simulink model "DDCU_wxt_v02_forA_LabviewV02"  (R2014a)
settings: Solver=FixedStepDiscrete  StartTime=0.0  StopTime=50  FixedStep=0.0005  RelTol=1e-3
InitFcn:
  | Veh_Par_wxt
values from neighbouring files (symbols this model uses):
  ag_thr = 0.4*g    (= 3.924)    [Veh_Par_wxt.m]
  B = 2.25    [Veh_Par_wxt.m]
  bra_pre_em = 12    [Veh_Par_wxt.m]
  bra_pre_gz2 = 12/3    (= 4)    [Veh_Par_wxt.m]
  bra_pre_gz34 = 12/3    (= 4)    [Veh_Par_wxt.m]
  bra_pre_yd = 12/2    (= 6)    [Veh_Par_wxt.m]
  brakepre_dem_data = [0 1 2 3 4 5 6 7 8 9 10 11 12]    [Veh_Par_wxt.m]
  brakeTrq_dem_data = [0 218.198 436.396 654.594 872.792 1090.99 1309.188 1527.386 1745.584 1963.782 2181.98 2400.178 2618.376]    [Veh_Par_wxt.m]
  bratrq_max = 4*2618.376    (= 10473.504)    [Veh_Par_wxt.m]
  eff_tran = 0.75    [Veh_Par_wxt.m]
  G = Mass*g    (= 36297)    [Veh_Par_wxt.m]
  kd1 = 1    [Veh_Par_wxt.m]
  kd2 = 1    [Veh_Par_wxt.m]
  kd3 = 1    [Veh_Par_wxt.m]
  ki1 = 1    [Veh_Par_wxt.m]
  ki2 = 1    [Veh_Par_wxt.m]
  ki3 = 1    [Veh_Par_wxt.m]
  kp1 = 1    [Veh_Par_wxt.m]
  kp2 = 1    [Veh_Par_wxt.m]
  kp3 = 1    [Veh_Par_wxt.m]
  L = 3.12    [Veh_Par_wxt.m]
  premax = 12    [Veh_Par_wxt.m]
  Radius = 0.20    (= 0.2)    [Veh_Par_wxt.m]
  s_opt_yi_add = 0.05    [Veh_Par_wxt.m]
  s_opt_zhuan_add = 0.05    [Veh_Par_wxt.m]
  spd_map_mot = [0 100 200 300 360 400 500 600 700 800 900]*tras_ratio    [Veh_Par_wxt.m]
  spdmax = 900*tras_ratio    (= 5580)    [Veh_Par_wxt.m]
  speed_thr_park = 5/3.6/Radius*30/pi    (= 66.3145596216)    [Veh_Par_wxt.m]
  tras_ratio = 6.2    [Veh_Par_wxt.m]
  trq_map_mot = [1200 1200 1200 1200 1200 1080 864 720 617 540 480]/tras_ratio    [Veh_Par_wxt.m]
  trqmax = 80    [Veh_Par_wxt.m]
  v_thr1_b = 5    [Veh_Par_wxt.m]
  v_thr2_b = 20    [Veh_Par_wxt.m]
  v_thr_park = 5    [Veh_Par_wxt.m]
undefined symbols (not defined in the file or in its folder): DiscIntNeverNeededParam
libraries: simulink x231, ec5744lib x19
(part 3 of 16)

== system DDCU_wxt_v02_forA_LabviewV02/OutputSignalProcess/VCU_MCU2 ==
  M3Enable_in : Inport
  M3Mode_in : Inport  Port=2
  M3Drive_in : Inport  Port=3
  M3TorqueSet_in : Inport  Port=4
  M3SpeedLimit_in : Inport  Port=5
  M4Enable_in : Inport  Port=6
  M4Mode_in : Inport  Port=7
  M4Drive_in : Inport  Port=8
  M4TorqueSet_in : Inport  Port=9
  M4SpeedLimit_in : Inport  Port=10
  MCU2HeartBeat_in : Inport  Port=11
  Conv{1..8} (8 alike) : DataTypeConversion
  M3Drive : Subsystem
  M3Enable : Subsystem
  M3Mode : Subsystem
  M3SpeedLimit : Subsystem
  M3TorqueSet : Subsystem
  M4Drive : Subsystem
  M4Enable : Subsystem
  M4Mode : Subsystem
  M4SpeedLimit : Subsystem
  M4TorqueSet : Subsystem
  MCU2HeartBeat : Subsystem
  VCU_MCU2_DLC : Constant  Value=8  OutDataTypeStr=uint8
  VCU_MCU2_DLC_Out : Terminator
  VCU_MCU2_ID : Constant  Value=2348937218  OutDataTypeStr=single
  VCU_MCU2_ID_Out : Terminator
  VCU_MCU2_mux : Mux  Inputs=8
  or{1..8} (8 alike) : simulink/Logic and Bit Operations/Bitwise Operator  logicop=OR  UseBitMask=off  NumInputPorts=11  BitMask=bin2dec('11011001')  BitMaskRealWorld=Stored Integer
  output : Outport
  wires:
  VCU_MCU2_mux/1 -> output/1
  MCU2HeartBeat/1(output1) -> or1/1
  MCU2HeartBeat/2(output2) -> or2/1
  MCU2HeartBeat/3(output3) -> or3/1
  MCU2HeartBeat/4(output4) -> or4/1
  MCU2HeartBeat/5(output5) -> or5/1
  MCU2HeartBeat/6(output6) -> or6/1
  MCU2HeartBeat/7(output7) -> or7/1
  MCU2HeartBeat/8(output8) -> or8/1
  M4TorqueSet/1(output1) -> or1/2
  M4TorqueSet/2(output2) -> or2/2
  M4TorqueSet/3(output3) -> or3/2
  M4TorqueSet/4(output4) -> or4/2
  M4TorqueSet/5(output5) -> or5/2
  M4TorqueSet/6(output6) -> or6/2
  M4TorqueSet/7(output7) -> or7/2
  M4TorqueSet/8(output8) -> or8/2
  M4SpeedLimit/1(output1) -> or1/3
  M4SpeedLimit/2(output2) -> or2/3
  M4SpeedLimit/3(output3) -> or3/3
  M4SpeedLimit/4(output4) -> or4/3
  M4SpeedLimit/5(output5) -> or5/3
  M4SpeedLimit/6(output6) -> or6/3
  M4SpeedLimit/7(output7) -> or7/3
  M4SpeedLimit/8(output8) -> or8/3
  M4Mode/1(output1) -> or1/4
  M4Mode/2(output2) -> or2/4
  M4Mode/3(output3) -> or3/4
  M4Mode/4(output4) -> or4/4
  M4Mode/5(output5) -> or5/4
  M4Mode/6(output6) -> or6/4
  M4Mode/7(output7) -> or7/4
  M4Mode/8(output8) -> or8/4
  M4Enable/1(output1) -> or1/5
  M4Enable/2(output2) -> or2/5
  M4Enable/3(output3) -> or3/5
  M4Enable/4(output4) -> or4/5
  M4Enable/5(output5) -> or5/5
  M4Enable/6(output6) -> or6/5
  M4Enable/7(output7) -> or7/5
  M4Enable/8(output8) -> or8/5
  M4Drive/1(output1) -> or1/6
  M4Drive/2(output2) -> or2/6
  M4Drive/3(output3) -> or3/6
  M4Drive/4(output4) -> or4/6
  M4Drive/5(output5) -> or5/6
  M4Drive/6(output6) -> or6/6
  M4Drive/7(output7) -> or7/6
  M4Drive/8(output8) -> or8/6
  M3TorqueSet/1(output1) -> or1/7
  M3TorqueSet/2(output2) -> or2/7
  M3TorqueSet/3(output3) -> or3/7
  M3TorqueSet/4(output4) -> or4/7
  M3TorqueSet/5(output5) -> or5/7
  M3TorqueSet/6(output6) -> or6/7
  M3TorqueSet/7(output7) -> or7/7
  M3TorqueSet/8(output8) -> or8/7
  M3SpeedLimit/1(output1) -> or1/8
  M3SpeedLimit/2(output2) -> or2/8
  M3SpeedLimit/3(output3) -> or3/8
  M3SpeedLimit/4(output4) -> or4/8
  M3SpeedLimit/5(output5) -> or5/8
  M3SpeedLimit/6(output6) -> or6/8
  M3SpeedLimit/7(output7) -> or7/8
  M3SpeedLimit/8(output8) -> or8/8
  M3Mode/1(output1) -> or1/9
  M3Mode/2(output2) -> or2/9
  M3Mode/3(output3) -> or3/9
  M3Mode/4(output4) -> or4/9
  M3Mode/5(output5) -> or5/9
  M3Mode/6(output6) -> or6/9
  M3Mode/7(output7) -> or7/9
  M3Mode/8(output8) -> or8/9
  M3Enable/1(output1) -> or1/10
  M3Enable/2(output2) -> or2/10
  M3Enable/3(output3) -> or3/10
  M3Enable/4(output4) -> or4/10
  M3Enable/5(output5) -> or5/10
  M3Enable/6(output6) -> or6/10
  M3Enable/7(output7) -> or7/10
  M3Enable/8(output8) -> or8/10
  M3Drive/1(output1) -> or1/11
  M3Drive/2(output2) -> or2/11
  M3Drive/3(output3) -> or3/11
  M3Drive/4(output4) -> or4/11
  M3Drive/5(output5) -> or5/11
  M3Drive/6(output6) -> or6/11
  M3Drive/7(output7) -> or7/11
  M3Drive/8(output8) -> or8/11
  or1/1 -> Conv1/1
  Conv1/1 -> VCU_MCU2_mux/1
  or2/1 -> Conv2/1
  Conv2/1 -> VCU_MCU2_mux/2
  or3/1 -> Conv3/1
  Conv3/1 -> VCU_MCU2_mux/3
  or4/1 -> Conv4/1
  Conv4/1 -> VCU_MCU2_mux/4
  or5/1 -> Conv5/1
  Conv5/1 -> VCU_MCU2_mux/5
  or6/1 -> Conv6/1
  Conv6/1 -> VCU_MCU2_mux/6
  or7/1 -> Conv7/1
  Conv7/1 -> VCU_MCU2_mux/7
  or8/1 -> Conv8/1
  Conv8/1 -> VCU_MCU2_mux/8
  VCU_MCU2_ID/1 -> VCU_MCU2_ID_Out/1
  VCU_MCU2_DLC/1 -> VCU_MCU2_DLC_Out/1
  MCU2HeartBeat_in/1 -> MCU2HeartBeat/1(MCU2HeartBeat)
  M4TorqueSet_in/1 -> M4TorqueSet/1(M4TorqueSet)
  M4SpeedLimit_in/1 -> M4SpeedLimit/1(M4SpeedLimit)
  M4Mode_in/1 -> M4Mode/1(M4Mode)
  M4Enable_in/1 -> M4Enable/1(M4Enable)
  M4Drive_in/1 -> M4Drive/1(M4Drive)
  M3TorqueSet_in/1 -> M3TorqueSet/1(M3TorqueSet)
  M3SpeedLimit_in/1 -> M3SpeedLimit/1(M3SpeedLimit)
  M3Mode_in/1 -> M3Mode/1(M3Mode)
  M3Enable_in/1 -> M3Enable/1(M3Enable)
  M3Drive_in/1 -> M3Drive/1(M3Drive)

== matlab function DDCU_wxt_v02_forA_LabviewV02/MainControl/mode_control/forward/forward/Drive/驱动防滑控制TCS/转向TCS/左转/前轮滑转/HeartBeat ==
  data: life_pre input; life output
function life = fcn(life_pre)
%#codegen
life=life_pre+1;
if life>15
    life=0;
end
end

== matlab function DDCU_wxt_v02_forA_LabviewV02/MainControl/mode_control/forward/forward/Drive/驱动防滑控制TCS/转向TCS/左转/后轮滑转/HeartBeat ==
  data: life_pre input; life output
function life = fcn(life_pre)
%#codegen
life=life_pre+1;
if life>15
    life=0;
end
end

== matlab function DDCU_wxt_v02_forA_LabviewV02/MainControl/mode_control/forward/forward/Drive/驱动防滑控制TCS/转向TCS/左转/前后轮均滑转/HeartBeat ==
  data: life_pre input; life output
function life = fcn(life_pre)
%#codegen
life=life_pre+1;
if life>15
    life=0;
end
end

== matlab function DDCU_wxt_v02_forA_LabviewV02/MainControl/mode_control/forward/forward/Drive/驱动防滑控制TCS/转向TCS/右转/MATLAB Function1 ==
  data: s_act_lr input; flag_lr output; s_opt_zhuan input; s_opt_zhuan_add input; flag_lr_pre input
function flag_lr = fcn(s_act_lr,s_opt_zhuan,s_opt_zhuan_add,flag_lr_pre)
%#codegen
if s_act_lr>s_opt_zhuan+s_opt_zhuan_add
    flag_lr=1;
elseif s_act_lr<s_opt_zhuan
    flag_lr = 0;
else
    flag_lr=flag_lr_pre;
end
end

== matlab function DDCU_wxt_v02_forA_LabviewV02/MainControl/mode_control/forward/forward/Drive/驱动防滑控制TCS/转向TCS/右转/MATLAB Function4 ==
  data: y output; flag_lf input; flag_lr input
function y = fcn(flag_lf,flag_lr)
%#codegen只判断外侧车轮滑转状况，不能满足要求再进一步修改。
if flag_lf==0 && flag_lr==0
    y=0;
elseif flag_lf==1 && flag_lr==0
    y=1;
elseif flag_lf==0 && flag_lr==1
    y=2;
else
    %     flag_lf==1 && flag_lr==1
    y=3;
end
end

== matlab function DDCU_wxt_v02_forA_LabviewV02/MainControl/mode_control/forward/forward/Drive/驱动防滑控制TCS/转向TCS/右转/后轮滑转/HeartBeat1 ==
  data: life_pre input; life output
function life = fcn(life_pre)
%#codegen
life=life_pre+1;
if life>15
    life=0;
end
end

== matlab function DDCU_wxt_v02_forA_LabviewV02/MainControl/mode_control/forward/forward/Drive/驱动防滑控制TCS/转向TCS/右转/无滑转/HeartBeat ==
  data: life_pre input; life output
function life = fcn(life_pre)
%#codegen
life=life_pre+1;
if life>15
    life=0;
end
end

== matlab function DDCU_wxt_v02_forA_LabviewV02/MainControl/mode_control/neutral/neutral/HeartBeat ==
  data: life_pre input; life output
function life = fcn(life_pre)
%#codegen
life=life_pre+1;
if life>15
    life=0;
end
end

== matlab function DDCU_wxt_v02_forA_LabviewV02/MainControl/mode_control/forward/forward/Brake/MATLAB Function2 ==
  data: syi_act_lr input; flagyi_lr output; s_opt_yi input; s_opt_yi_add input; flagyi_lr_pre input
function flagyi_lr = fcn(syi_act_lr,s_opt_yi,s_opt_yi_add,flagyi_lr_pre)
%#codegen
if syi_act_lr>s_opt_yi+s_opt_yi_add
    flagyi_lr=1;
elseif syi_act_lr<s_opt_yi
    flagyi_lr = 0;
else
    flagyi_lr=flagyi_lr_pre;
end
end

== matlab function DDCU_wxt_v02_forA_LabviewV02/MainControl/mode_control/forward/forward/Brake/HeartBeat ==
  data: life_pre input; life output
function life = fcn(life_pre)
%#codegen
life=life_pre+1;
if life>15
    life=0;
end
end

== matlab function DDCU_wxt_v02_forA_LabviewV02/MainControl/mode_control/center_steer/center_steer/容错控制/MATLAB Function ==
  data: trq_dem_l input; trq_dem_lf output; trq_dem_r input; trqlim_lf input; trqlim_lr input; trqlim_rf input; trqlim_rr input; guzhang_lf input; guzhang_lr input; guzhang_rf input; guzhang_rr input; trq_dem_lr output; trq_dem_rf output; trq_dem_rr output; bra_pre_l output; bra_pre_r output; bra_pre_yd input; mode output
function [trq_dem_lf,trq_dem_lr,trq_dem_rf,trq_dem_rr,bra_pre_l,bra_pre_r,mode] = fcn(trq_dem_l,trq_dem_r,trqlim_lf,trqlim_lr,trqlim_rf,trqlim_rr,guzhang_lf,guzhang_lr,guzhang_rf,guzhang_rr,bra_pre_yd)
%#codegen
if guzhang_lf==0 && guzhang_lr==0 && guzhang_rf==0 && guzhang_rr==0    %0电机故障,平均分配
    trq_dem_lf=trq_dem_l/2;
    trq_dem_lr=trq_dem_l/2;
    trq_dem_rf=trq_dem_r/2;
    trq_dem_rr=trq_dem_r/2;
    bra_pre_l=0;
    bra_pre_r=0;
    mode=1;
elseif  guzhang_lf==1 && guzhang_lr==0 && guzhang_rf==0 && guzhang_rr==0  %1电机故障，同侧电机进行力矩转移,跟行车不同，对侧不降扭。
    trq_dem_lf=0;
    trq_dem_lr=min(trq_dem_l,trqlim_lr);
    trq_dem_rf=trq_dem_r/2;
    trq_dem_rr=trq_dem_r/2;
    bra_pre_l=0;
    bra_pre_r=0;
    mode=2;
elseif  guzhang_lf==0 && guzhang_lr==1 && guzhang_rf==0 && guzhang_rr==0
    trq_dem_lf=min(trq_dem_l,trqlim_lf);
    trq_dem_lr=0;
    trq_dem_rf=trq_dem_r/2;
    trq_dem_rr=trq_dem_r/2;
    bra_pre_l=0;
    bra_pre_r=0;
    mode=3;
elseif  guzhang_lf==0 && guzhang_lr==0 && guzhang_rf==1 && guzhang_rr==0
    trq_dem_rf=0;
    trq_dem_rr=min(trq_dem_r,trqlim_rr);
    trq_dem_lf=trq_dem_l/2;
    trq_dem_lr=trq_dem_l/2;
    bra_pre_l=0;
    bra_pre_r=0;
    mode=4;
elseif  guzhang_lf==0 && guzhang_lr==0 && guzhang_rf==0 && guzhang_rr==1
    trq_dem_rf=min(trq_dem_r,trqlim_rf);
    trq_dem_rr=0;
    trq_dem_lf=trq_dem_l/2;
    trq_dem_lr=trq_dem_l/2;
    bra_pre_l=0;
    bra_pre_r=0;
    mode=5;
elseif  guzhang_lf==1 && guzhang_lr==1 && guzhang_rf==0 && guzhang_rr==0  %2电机故障，左侧双电机故障，左侧履带施加制动，改为原地转向
    trq_dem_lf=0;
    trq_dem_lr=0;
    trq_dem_rf=trq_dem_r/2;
    trq_dem_rr=trq_dem_r/2;
    bra_pre_l=bra_pre_yd;
    bra_pre_r=0;
    mode=6;
elseif  guzhang_lf==0 && guzhang_lr==0 && guzhang_rf==1 && guzhang_rr==1  %右侧双电机故障
    trq_dem_lf=trq_dem_l/2;
    trq_dem_lr=trq_dem_l/2;
    trq_dem_rf=0;
    trq_dem_rr=0;
    bra_pre_l=0;
    bra_pre_r=bra_pre_yd;
    mode=7;
elseif  guzhang_lf==1 && guzhang_lr==0 && guzhang_rf==1 && guzhang_rr==0 %2电机故障，对侧双电机故障,有4种情况,前两电机故障
    trq_dem_lf=0;
    trq_dem_rf=0;
    trq_dem_lr=min(trq_dem_l,trqlim_lr);
    trq_dem_rr=min(trq_dem_r,trqlim_rr);
    bra_pre_l=0;
    bra_pre_r=0;
    mode=8;
elseif  guzhang_lf==0 && guzhang_lr==1 && guzhang_rf==0 && guzhang_rr==1 %后两电机故障
    trq_dem_lr=0;
    trq_dem_rr=0;
    trq_dem_lf=min(trq_dem_l,trqlim_lf);
    trq_dem_rf=min(trq_dem_r,trqlim_rf);
    bra_pre_l=0;
    bra_pre_r=0;
    mode=9;
elseif  guzhang_lf==1 && guzhang_lr==0 && guzhang_rf==0 && guzhang_rr==1 %左前电机和右后电机故障
    trq_dem_lf=0;
    trq_dem_rr=0;
    trq_dem_lr=min(trq_dem_l,trqlim_lr);
    trq_dem_rf=min(trq_dem_r,trqlim_rf);
    bra_pre_l=0;
    bra_pre_r=0;
    mode=10;
elseif  guzhang_lf==0 && guzhang_lr==1 && guzhang_rf==1 && guzhang_rr==0 %左后电机和右前电机故障
    trq_dem_lr=0;
    trq_dem_rf=0;
    trq_dem_lf=min(trq_dem_l,trqlim_lf);
    trq_dem_rr=min(trq_dem_r,trqlim_rr);
    bra_pre_l=0;
    bra_pre_r=0;
    mode=11;
elseif guzhang_lf==1 && guzhang_lr==1 && guzhang_rf==1 && guzhang_rr==0   % 三电机故障
    trq_dem_lf=0;
    trq_dem_lr=0;
    trq_dem_rf=0;
    trq_dem_rr=min(trq_dem_r,trqlim_rr);
    bra_pre_l=bra_pre_yd;
    bra_pre_r=0;
    mode=12;
elseif guzhang_lf==1 && guzhang_lr==1 && guzhang_rf==0 && guzhang_rr==1
    trq_dem_lf=0;
    trq_dem_lr=0;
    trq_dem_rf=min(trq_dem_r,trqlim_rf);
    trq_dem_rr=0;
    bra_pre_l=bra_pre_yd;
    bra_pre_r=0;
    mode=13;
elseif guzhang_lf==1 && guzhang_lr==0 && guzhang_rf==1 && guzhang_rr==1
    trq_dem_lf=0;
    trq_dem_lr=min(trq_dem_l,trqlim_lr);
    trq_dem_rf=0;
    trq_dem_rr=0;
    bra_pre_l=0;
    bra_pre_r=bra_pre_yd;
    mode=14;
elseif guzhang_lf==0 && guzhang_lr==1 && guzhang_rf==1 && guzhang_rr==1
    trq_dem_lf=min(trq_dem_l,trqlim_lf);
    trq_dem_lr=0;
    trq_dem_rf=0;
    trq_dem_rr=0;
    bra_pre_l=0;
    bra_pre_r=bra_pre_yd;
    mode=15;
else
    %     guzhang_lf==1 && guzhang_lr==1 && guzhang_rf==1 && guzhang_rr==1 %四电机故障
    trq_dem_lf=0;
    trq_dem_lr=0;
    trq_dem_rf=0;
    trq_dem_rr=0;
    bra_pre_l=0;
    bra_pre_r=0;
    mode=16;
end
trq_dem_lf=min(trqlim_lf,trq_dem_lf);trq_dem_lf=max(0,trq_dem_lf);
trq_dem_lr=min(trqlim_lr,trq_dem_lr);trq_dem_lr=max(0,trq_dem_lr);
trq_dem_rf=min(trqlim_rf,trq_dem_rf);trq_dem_rf=max(0,trq_dem_rf);
trq_dem_rr=min(trqlim_rr,trq_dem_rr);trq_dem_rr=max(0,trq_dem_rr);
bra_pre_l=bra_pre_l;
bra_pre_r=bra_pre_r;
end

== system DDCU_wxt_v02_forA_LabviewV02/OutputSignalProcess/VCU_MCU2_replace ==
  M4SpeedSet_in : Inport
  M3SpeedSet_in : Inport  Port=2
  MCU2HeartBeat_in : Inport  Port=3
  M4SpeedLimit_in : Inport  Port=4
  M4Mode_in : Inport  Port=5
  M4Enable_in : Inport  Port=6
  M4Drive_in : Inport  Port=7
  M3SpeedLimit_in : Inport  Port=8
  M3Mode_in : Inport  Port=9
  M3Enable_in : Inport  Port=10
  M3Drive_in : Inport  Port=11
  Conv{1..8} (8 alike) : DataTypeConversion
  M3Drive : Subsystem
  M3Enable : Subsystem
  M3Mode : Subsystem
  M3SpeedLimit : Subsystem
  M3SpeedSet : Subsystem
  M4Drive : Subsystem
  M4Enable : Subsystem
  M4Mode : Subsystem
  M4SpeedLimit : Subsystem
  M4SpeedSet : Subsystem
  MCU2HeartBeat : Subsystem
  VCU_MCU2_replace_DLC : Constant  Value=8  OutDataTypeStr=uint8
  VCU_MCU2_replace_DLC_Out : Terminator
  VCU_MCU2_replace_ID : Constant  Value=2348937234  OutDataTypeStr=single
  VCU_MCU2_replace_ID_Out : Terminator
  VCU_MCU2_replace_mux : Mux  Inputs=8
  or{1..8} (8 alike) : simulink/Logic and Bit Operations/Bitwise Operator  logicop=OR  UseBitMask=off  NumInputPorts=11  BitMask=bin2dec('11011001')  BitMaskRealWorld=Stored Integer
  output : Outport
  wires:
  VCU_MCU2_replace_mux/1 -> output/1
  M4SpeedSet/1(output1) -> or1/1
  M4SpeedSet/2(output2) -> or2/1
  M4SpeedSet/3(output3) -> or3/1
  M4SpeedSet/4(output4) -> or4/1
  M4SpeedSet/5(output5) -> or5/1
  M4SpeedSet/6(output6) -> or6/1
  M4SpeedSet/7(output7) -> or7/1
  M4SpeedSet/8(output8) -> or8/1
  M3SpeedSet/1(output1) -> or1/2
  M3SpeedSet/2(output2) -> or2/2
  M3SpeedSet/3(output3) -> or3/2
  M3SpeedSet/4(output4) -> or4/2
  M3SpeedSet/5(output5) -> or5/2
  M3SpeedSet/6(output6) -> or6/2
  M3SpeedSet/7(output7) -> or7/2
  M3SpeedSet/8(output8) -> or8/2
  MCU2HeartBeat/1(output1) -> or1/3
  MCU2HeartBeat/2(output2) -> or2/3
  MCU2HeartBeat/3(output3) -> or3/3
  MCU2HeartBeat/4(output4) -> or4/3
  MCU2HeartBeat/5(output5) -> or5/3
  MCU2HeartBeat/6(output6) -> or6/3
  MCU2HeartBeat/7(output7) -> or7/3
  MCU2HeartBeat/8(output8) -> or8/3
  M4SpeedLimit/1(output1) -> or1/4
  M4SpeedLimit/2(output2) -> or2/4
  M4SpeedLimit/3(output3) -> or3/4
  M4SpeedLimit/4(output4) -> or4/4
  M4SpeedLimit/5(output5) -> or5/4
  M4SpeedLimit/6(output6) -> or6/4
  M4SpeedLimit/7(output7) -> or7/4
  M4SpeedLimit/8(output8) -> or8/4
  M4Mode/1(output1) -> or1/5
  M4Mode/2(output2) -> or2/5
  M4Mode/3(output3) -> or3/5
  M4Mode/4(output4) -> or4/5
  M4Mode/5(output5) -> or5/5
  M4Mode/6(output6) -> or6/5
  M4Mode/7(output7) -> or7/5
  M4Mode/8(output8) -> or8/5
  M4Enable/1(output1) -> or1/6
  M4Enable/2(output2) -> or2/6
  M4Enable/3(output3) -> or3/6
  M4Enable/4(output4) -> or4/6
  M4Enable/5(output5) -> or5/6
  M4Enable/6(output6) -> or6/6
  M4Enable/7(output7) -> or7/6
  M4Enable/8(output8) -> or8/6
  M4Drive/1(output1) -> or1/7
  M4Drive/2(output2) -> or2/7
  M4Drive/3(output3) -> or3/7
  M4Drive/4(output4) -> or4/7
  M4Drive/5(output5) -> or5/7
  M4Drive/6(output6) -> or6/7
  M4Drive/7(output7) -> or7/7
  M4Drive/8(output8) -> or8/7
  M3SpeedLimit/1(output1) -> or1/8
  M3SpeedLimit/2(output2) -> or2/8
  M3SpeedLimit/3(output3) -> or3/8
  M3SpeedLimit/4(output4) -> or4/8
  M3SpeedLimit/5(output5) -> or5/8
  M3SpeedLimit/6(output6) -> or6/8
  M3SpeedLimit/7(output7) -> or7/8
  M3SpeedLimit/8(output8) -> or8/8
  M3Mode/1(output1) -> or1/9
  M3Mode/2(output2) -> or2/9
  M3Mode/3(output3) -> or3/9
  M3Mode/4(output4) -> or4/9
  M3Mode/5(output5) -> or5/9
  M3Mode/6(output6) -> or6/9
  M3Mode/7(output7) -> or7/9
  M3Mode/8(output8) -> or8/9
  M3Enable/1(output1) -> or1/10
  M3Enable/2(output2) -> or2/10
  M3Enable/3(output3) -> or3/10
  M3Enable/4(output4) -> or4/10
  M3Enable/5(output5) -> or5/10
  M3Enable/6(output6) -> or6/10
  M3Enable/7(output7) -> or7/10
  M3Enable/8(output8) -> or8/10
  M3Drive/1(output1) -> or1/11
  M3Drive/2(output2) -> or2/11
  M3Drive/3(output3) -> or3/11
  M3Drive/4(output4) -> or4/11
  M3Drive/5(output5) -> or5/11
  M3Drive/6(output6) -> or6/11
  M3Drive/7(output7) -> or7/11
  M3Drive/8(output8) -> or8/11
  or1/1 -> Conv1/1
  Conv1/1 -> VCU_MCU2_replace_mux/1
  or2/1 -> Conv2/1
  Conv2/1 -> VCU_MCU2_replace_mux/2
  or3/1 -> Conv3/1
  Conv3/1 -> VCU_MCU2_replace_mux/3
  or4/1 -> Conv4/1
  Conv4/1 -> VCU_MCU2_replace_mux/4
  or5/1 -> Conv5/1
  Conv5/1 -> VCU_MCU2_replace_mux/5
  or6/1 -> Conv6/1
  Conv6/1 -> VCU_MCU2_replace_mux/6
  or7/1 -> Conv7/1
  Conv7/1 -> VCU_MCU2_replace_mux/7
  or8/1 -> Conv8/1
  Conv8/1 -> VCU_MCU2_replace_mux/8
  VCU_MCU2_replace_ID/1 -> VCU_MCU2_replace_ID_Out/1
  VCU_MCU2_replace_DLC/1 -> VCU_MCU2_replace_DLC_Out/1
  M4SpeedSet_in/1 -> M4SpeedSet/1(M4SpeedSet)
  M3SpeedSet_in/1 -> M3SpeedSet/1(M3SpeedSet)
  MCU2HeartBeat_in/1 -> MCU2HeartBeat/1(MCU2HeartBeat)
  M4SpeedLimit_in/1 -> M4SpeedLimit/1(M4SpeedLimit)
  M4Mode_in/1 -> M4Mode/1(M4Mode)
  M4Enable_in/1 -> M4Enable/1(M4Enable)
  M4Drive_in/1 -> M4Drive/1(M4Drive)
  M3SpeedLimit_in/1 -> M3SpeedLimit/1(M3SpeedLimit)
  M3Mode_in/1 -> M3Mode/1(M3Mode)
  M3Enable_in/1 -> M3Enable/1(M3Enable)
  M3Drive_in/1 -> M3Drive/1(M3Drive)

== system DDCU_wxt_v02_forA_LabviewV02/OutputSignalProcess/VCU_Park ==
  ParkEnable_in : Inport
  Conv{1..8} (8 alike) : DataTypeConversion
  ParkEnable : Subsystem
  VCU_Park_DLC : Constant  Value=8  OutDataTypeStr=uint8
  VCU_Park_DLC_Out : Terminator
  VCU_Park_ID : Constant  Value=2281988666  OutDataTypeStr=single
  VCU_Park_ID_Out : Terminator
  VCU_Park_mux : Mux  Inputs=8
  or{1..8} (8 alike) : simulink/Logic and Bit Operations/Bitwise Operator  logicop=OR  UseBitMask=off  BitMask=bin2dec('11011001')  BitMaskRealWorld=Stored Integer
  output : Outport
  wires:
  VCU_Park_mux/1 -> output/1
  ParkEnable/1(output1) -> or1/1
  ParkEnable/2(output2) -> or2/1
  ParkEnable/3(output3) -> or3/1
  ParkEnable/4(output4) -> or4/1
  ParkEnable/5(output5) -> or5/1
  ParkEnable/6(output6) -> or6/1
  ParkEnable/7(output7) -> or7/1
  ParkEnable/8(output8) -> or8/1
  or1/1 -> Conv1/1
  Conv1/1 -> VCU_Park_mux/1
  or2/1 -> Conv2/1
  Conv2/1 -> VCU_Park_mux/2
  or3/1 -> Conv3/1
  Conv3/1 -> VCU_Park_mux/3
  or4/1 -> Conv4/1
  Conv4/1 -> VCU_Park_mux/4
  or5/1 -> Conv5/1
  Conv5/1 -> VCU_Park_mux/5
  or6/1 -> Conv6/1
  Conv6/1 -> VCU_Park_mux/6
  or7/1 -> Conv7/1
  Conv7/1 -> VCU_Park_mux/7
  or8/1 -> Conv8/1
  Conv8/1 -> VCU_Park_mux/8
  VCU_Park_ID/1 -> VCU_Park_ID_Out/1
  VCU_Park_DLC/1 -> VCU_Park_DLC_Out/1
  ParkEnable_in/1 -> ParkEnable/1(ParkEnable)

== system DDCU_wxt_v02_forA_LabviewV02/Data_Input/Function-Call Subsystem/ddcu1_ddcu2 ==
  input : Inport
  Enable : EnablePort
  Demux : Demux  Outputs=8
  acc_dem_Ad : Sum
  acc_dem_Convert : DataTypeConversion  OutDataTypeStr=uint32
  acc_dem_F : Gain
  acc_dem_L : simulink/Logic and Bit Operations/Bitwise Operator  logicop=AND  UseBitMask=on  BitMask=255  BitMaskRealWorld=Stored Integer
  acc_dem_O : Constant  Value=0  OutDataTypeStr=single
  acc_dem_S : ArithShift
  acc_dem_Sub : Subsystem
  acc_dem_sat : Saturate  UpperLimit=255  LowerLimit=0
  acc_demcv : DataTypeConversion
  brake_dem_Ad : Sum
  brake_dem_Convert : DataTypeConversion  OutDataTypeStr=uint32
  brake_dem_F : Gain
  brake_dem_L : simulink/Logic and Bit Operations/Bitwise Operator  logicop=AND  UseBitMask=on  BitMask=255  BitMaskRealWorld=Stored Integer
  brake_dem_O : Constant  Value=0  OutDataTypeStr=single
  brake_dem_S : ArithShift
  brake_dem_Sub : Subsystem
  brake_dem_sat : Saturate  UpperLimit=255  LowerLimit=0
  brake_demcv : DataTypeConversion
  brake_emerg_Ad : Sum
  brake_emerg_Convert : DataTypeConversion  OutDataTypeStr=uint32
  brake_emerg_F : Gain
  brake_emerg_L : simulink/Logic and Bit Operations/Bitwise Operator  logicop=AND  UseBitMask=on  BitMask=8  BitMaskRealWorld=Stored Integer
  brake_emerg_O : Constant  Value=0  OutDataTypeStr=single
  brake_emerg_S : ArithShift  BitShiftNumber=3
  brake_emerg_Sub : Subsystem
  brake_emerg_sat : Saturate  UpperLimit=1  LowerLimit=0
  brake_emergcv : DataTypeConversion
  mode_dem_Ad : Sum
  mode_dem_Convert : DataTypeConversion  OutDataTypeStr=uint32
  mode_dem_F : Gain
  mode_dem_L : simulink/Logic and Bit Operations/Bitwise Operator  logicop=AND  UseBitMask=on  BitMask=7  BitMaskRealWorld=Stored Integer
  mode_dem_O : Constant  Value=0  OutDataTypeStr=single
  mode_dem_S : ArithShift
  mode_dem_Sub : Subsystem
  mode_dem_sat : Saturate  UpperLimit=7  LowerLimit=0
  mode_demcv : DataTypeConversion
  steer_dem_Ad : Sum
  steer_dem_Convert : DataTypeConversion  OutDataTypeStr=uint32
  steer_dem_F : Gain
  steer_dem_L : simulink/Logic and Bit Operations/Bitwise Operator  logicop=AND  UseBitMask=on  BitMask=255  BitMaskRealWorld=Stored Integer
  steer_dem_O : Constant  Value=-100  OutDataTypeStr=single
  steer_dem_S : ArithShift
  steer_dem_Sub : Subsystem
  steer_dem_sat : Saturate  UpperLimit=155  LowerLimit=-100
  steer_demcv : DataTypeConversion
  brake_emerg_Out : Outport
  steer_dem_Out : Outport  Port=2
  mode_dem_Out : Outport  Port=3
  brake_dem_Out : Outport  Port=4
  acc_dem_Out : Outport  Port=5
  wires:
  brake_emerg_F/1 -> brake_emerg_Ad/1
  brake_emerg_O/1 -> brake_emerg_Ad/2
  brake_emerg_Ad/1 -> brake_emerg_sat/1
  brake_emerg_sat/1 -> brake_emerg_Out/1
  Demux/1 -> brake_emerg_Sub/1(In1), mode_dem_Sub/1(In1)
  brake_emerg_Sub/1(Out1) -> brake_emerg_Convert/1
  brake_emerg_Convert/1 -> brake_emerg_L/1
  brake_emerg_L/1 -> brake_emerg_S/1
  brake_emerg_S/1 -> brake_emergcv/1
  brake_emergcv/1 -> brake_emerg_F/1
  steer_dem_F/1 -> steer_dem_Ad/1
  steer_dem_O/1 -> steer_dem_Ad/2
  steer_dem_Ad/1 -> steer_dem_sat/1
  steer_dem_sat/1 -> steer_dem_Out/1
  Demux/3 -> steer_dem_Sub/1(In1)
  steer_dem_Sub/1(Out1) -> steer_dem_Convert/1
  steer_dem_Convert/1 -> steer_dem_L/1
  steer_dem_L/1 -> steer_dem_S/1
  steer_dem_S/1 -> steer_demcv/1
  steer_demcv/1 -> steer_dem_F/1
  mode_dem_F/1 -> mode_dem_Ad/1
  mode_dem_O/1 -> mode_dem_Ad/2
  mode_dem_Ad/1 -> mode_dem_sat/1
  mode_dem_sat/1 -> mode_dem_Out/1
  mode_dem_Sub/1(Out1) -> mode_dem_Convert/1
  mode_dem_Convert/1 -> mode_dem_L/1
  mode_dem_L/1 -> mode_dem_S/1
  mode_dem_S/1 -> mode_demcv/1
  mode_demcv/1 -> mode_dem_F/1
  brake_dem_F/1 -> brake_dem_Ad/1
  brake_dem_O/1 -> brake_dem_Ad/2
  brake_dem_Ad/1 -> brake_dem_sat/1
  brake_dem_sat/1 -> brake_dem_Out/1
  Demux/4 -> brake_dem_Sub/1(In1)
  brake_dem_Sub/1(Out1) -> brake_dem_Convert/1
  brake_dem_Convert/1 -> brake_dem_L/1
  brake_dem_L/1 -> brake_dem_S/1
  brake_dem_S/1 -> brake_demcv/1
  brake_demcv/1 -> brake_dem_F/1
  acc_dem_F/1 -> acc_dem_Ad/1
  acc_dem_O/1 -> acc_dem_Ad/2
  acc_dem_Ad/1 -> acc_dem_sat/1
  acc_dem_sat/1 -> acc_dem_Out/1
  Demux/2 -> acc_dem_Sub/1(In1)
  acc_dem_Sub/1(Out1) -> acc_dem_Convert/1
  acc_dem_Convert/1 -> acc_dem_L/1
  acc_dem_L/1 -> acc_dem_S/1
  acc_dem_S/1 -> acc_demcv/1
  acc_demcv/1 -> acc_dem_F/1
  input/1 -> Demux/1

== system DDCU_wxt_v02_forA_LabviewV02/Data_Input/Function-Call Subsystem1/ESC_VCU ==
  input : Inport
  Enable : EnablePort
  Demux : Demux  Outputs=8
  VESC_BrkFlt_enum_Ad : Sum
  VESC_BrkFlt_enum_Convert : DataTypeConversion  OutDataTypeStr=uint32
  VESC_BrkFlt_enum_F : Gain
  VESC_BrkFlt_enum_L : simulink/Logic and Bit Operations/Bitwise Operator  logicop=AND  UseBitMask=on  BitMask=255  BitMaskRealWorld=Stored Integer
  VESC_BrkFlt_enum_O : Constant  Value=0  OutDataTypeStr=single
  VESC_BrkFlt_enum_S : ArithShift
  VESC_BrkFlt_enum_Sub : Subsystem
  VESC_BrkFlt_enum_sat : Saturate  UpperLimit=255  LowerLimit=0
  VESC_BrkFlt_enumcv : DataTypeConversion
  VESC_BrkPLe_MPa_Ad : Sum
  VESC_BrkPLe_MPa_Convert : DataTypeConversion  OutDataTypeStr=uint32
  VESC_BrkPLe_MPa_F : Gain  Gain=0.1
  VESC_BrkPLe_MPa_L : simulink/Logic and Bit Operations/Bitwise Operator  logicop=AND  UseBitMask=on  BitMask=255  BitMaskRealWorld=Stored Integer
  VESC_BrkPLe_MPa_O : Constant  Value=0  OutDataTypeStr=single
  VESC_BrkPLe_MPa_S : ArithShift
  VESC_BrkPLe_MPa_Sub : Subsystem
  VESC_BrkPLe_MPa_sat : Saturate  UpperLimit=25.5  LowerLimit=0
  VESC_BrkPLe_MPacv : DataTypeConversion
  VESC_BrkPMa_MPa_Ad : Sum
  VESC_BrkPMa_MPa_Convert : DataTypeConversion  OutDataTypeStr=uint32
  VESC_BrkPMa_MPa_F : Gain  Gain=0.1
  VESC_BrkPMa_MPa_L : simulink/Logic and Bit Operations/Bitwise Operator  logicop=AND  UseBitMask=on  BitMask=255  BitMaskRealWorld=Stored Integer
  VESC_BrkPMa_MPa_O : Constant  Value=0  OutDataTypeStr=single
  VESC_BrkPMa_MPa_S : ArithShift
  VESC_BrkPMa_MPa_Sub : Subsystem
  VESC_BrkPMa_MPa_sat : Saturate  UpperLimit=25.5  LowerLimit=0
  VESC_BrkPMa_MPacv : DataTypeConversion
  VESC_BrkPRi_MPa_Ad : Sum
  VESC_BrkPRi_MPa_Convert : DataTypeConversion  OutDataTypeStr=uint32
  VESC_BrkPRi_MPa_F : Gain  Gain=0.1
  VESC_BrkPRi_MPa_L : simulink/Logic and Bit Operations/Bitwise Operator  logicop=AND  UseBitMask=on  BitMask=255  BitMaskRealWorld=Stored Integer
  VESC_BrkPRi_MPa_O : Constant  Value=0  OutDataTypeStr=single
  VESC_BrkPRi_MPa_S : ArithShift
  VESC_BrkPRi_MPa_Sub : Subsystem
  VESC_BrkPRi_MPa_sat : Saturate  UpperLimit=25.5  LowerLimit=0
  VESC_BrkPRi_MPacv : DataTypeConversion
  VESC_BrkPSetLe_MPa_Ad : Sum
  VESC_BrkPSetLe_MPa_Convert : DataTypeConversion  OutDataTypeStr=uint32
  VESC_BrkPSetLe_MPa_F : Gain  Gain=0.1
  VESC_BrkPSetLe_MPa_L : simulink/Logic and Bit Operations/Bitwise Operator  logicop=AND  UseBitMask=on  BitMask=255  BitMaskRealWorld=Stored Integer
  VESC_BrkPSetLe_MPa_O : Constant  Value=0  OutDataTypeStr=single
  VESC_BrkPSetLe_MPa_S : ArithShift
  VESC_BrkPSetLe_MPa_Sub : Subsystem
  VESC_BrkPSetLe_MPa_sat : Saturate  UpperLimit=25.5  LowerLimit=0
  VESC_BrkPSetLe_MPacv : DataTypeConversion
  VESC_BrkPSetRi_MPa_Ad : Sum
  VESC_BrkPSetRi_MPa_Convert : DataTypeConversion  OutDataTypeStr=uint32
  VESC_BrkPSetRi_MPa_F : Gain  Gain=0.1
  VESC_BrkPSetRi_MPa_L : simulink/Logic and Bit Operations/Bitwise Operator  logicop=AND  UseBitMask=on  BitMask=255  BitMaskRealWorld=Stored Integer
  VESC_BrkPSetRi_MPa_O : Constant  Value=0  OutDataTypeStr=single
  VESC_BrkPSetRi_MPa_S : ArithShift
  VESC_BrkPSetRi_MPa_Sub : Subsystem
  VESC_BrkPSetRi_MPa_sat : Saturate  UpperLimit=25.5  LowerLimit=0
  VESC_BrkPSetRi_MPacv : DataTypeConversion
  VESC_BrkReq_flg_Ad : Sum
  VESC_BrkReq_flg_Convert : DataTypeConversion  OutDataTypeStr=uint32
  VESC_BrkReq_flg_F : Gain
  VESC_BrkReq_flg_L : simulink/Logic and Bit Operations/Bitwise Operator  logicop=AND  UseBitMask=on  BitMask=64  BitMaskRealWorld=Stored Integer
  VESC_BrkReq_flg_O : Constant  Value=0  OutDataTypeStr=single
  VESC_BrkReq_flg_S : ArithShift  BitShiftNumber=6
  VESC_BrkReq_flg_Sub : Subsystem
  VESC_BrkReq_flg_sat : Saturate  UpperLimit=1  LowerLimit=0
  VESC_BrkReq_flgcv : DataTypeConversion
  VESC_HotSts_flg_Ad : Sum
  VESC_HotSts_flg_Convert : DataTypeConversion  OutDataTypeStr=uint32
  VESC_HotSts_flg_F : Gain
  VESC_HotSts_flg_L : simulink/Logic and Bit Operations/Bitwise Operator  logicop=AND  UseBitMask=on  BitMask=32  BitMaskRealWorld=Stored Integer
  VESC_HotSts_flg_O : Constant  Value=0  OutDataTypeStr=single
  VESC_HotSts_flg_S : ArithShift  BitShiftNumber=5
  VESC_HotSts_flg_Sub : Subsystem
  VESC_HotSts_flg_sat : Saturate  UpperLimit=1  LowerLimit=0
  VESC_HotSts_flgcv : DataTypeConversion
  VESC_ParkReq_flg_Ad : Sum
  VESC_ParkReq_flg_Convert : DataTypeConversion  OutDataTypeStr=uint32
  VESC_ParkReq_flg_F : Gain
  VESC_ParkReq_flg_L : simulink/Logic and Bit Operations/Bitwise Operator  logicop=AND  UseBitMask=on  BitMask=128  BitMaskRealWorld=Stored Integer
  VESC_ParkReq_flg_O : Constant  Value=0  OutDataTypeStr=single
  VESC_ParkReq_flg_S : ArithShift  BitShiftNumber=7
  VESC_ParkReq_flg_Sub : Subsystem
  VESC_ParkReq_flg_sat : Saturate  UpperLimit=1  LowerLimit=0
  VESC_ParkReq_flgcv : DataTypeConversion
  VESC_BrkPMa_MPa_Out : Outport
  VESC_BrkPSetRi_MPa_Out : Outport  Port=2
  VESC_BrkPSetLe_MPa_Out : Outport  Port=3
  VESC_BrkFlt_enum_Out : Outport  Port=4
  VESC_HotSts_flg_Out : Outport  Port=5
  VESC_BrkReq_flg_Out : Outport  Port=6
  VESC_ParkReq_flg_Out : Outport  Port=7
  VESC_BrkPRi_MPa_Out : Outport  Port=8
  VESC_BrkPLe_MPa_Out : Outport  Port=9
  wires:
  VESC_BrkPMa_MPa_F/1 -> VESC_BrkPMa_MPa_Ad/1
  VESC_BrkPMa_MPa_O/1 -> VESC_BrkPMa_MPa_Ad/2
  VESC_BrkPMa_MPa_Ad/1 -> VESC_BrkPMa_MPa_sat/1
  VESC_BrkPMa_MPa_sat/1 -> VESC_BrkPMa_MPa_Out/1
  Demux/7 -> VESC_BrkPMa_MPa_Sub/1(In1)
  VESC_BrkPMa_MPa_Sub/1(Out1) -> VESC_BrkPMa_MPa_Convert/1
  VESC_BrkPMa_MPa_Convert/1 -> VESC_BrkPMa_MPa_L/1
  VESC_BrkPMa_MPa_L/1 -> VESC_BrkPMa_MPa_S/1
  VESC_BrkPMa_MPa_S/1 -> VESC_BrkPMa_MPacv/1
  VESC_BrkPMa_MPacv/1 -> VESC_BrkPMa_MPa_F/1
  VESC_BrkPSetRi_MPa_F/1 -> VESC_BrkPSetRi_MPa_Ad/1
  VESC_BrkPSetRi_MPa_O/1 -> VESC_BrkPSetRi_MPa_Ad/2
  VESC_BrkPSetRi_MPa_Ad/1 -> VESC_BrkPSetRi_MPa_sat/1
  VESC_BrkPSetRi_MPa_sat/1 -> VESC_BrkPSetRi_MPa_Out/1
  Demux/6 -> VESC_BrkPSetRi_MPa_Sub/1(In1)
  VESC_BrkPSetRi_MPa_Sub/1(Out1) -> VESC_BrkPSetRi_MPa_Convert/1
  VESC_BrkPSetRi_MPa_Convert/1 -> VESC_BrkPSetRi_MPa_L/1
  VESC_BrkPSetRi_MPa_L/1 -> VESC_BrkPSetRi_MPa_S/1
  VESC_BrkPSetRi_MPa_S/1 -> VESC_BrkPSetRi_MPacv/1
  VESC_BrkPSetRi_MPacv/1 -> VESC_BrkPSetRi_MPa_F/1
  VESC_BrkPSetLe_MPa_F/1 -> VESC_BrkPSetLe_MPa_Ad/1
  VESC_BrkPSetLe_MPa_O/1 -> VESC_BrkPSetLe_MPa_Ad/2
  VESC_BrkPSetLe_MPa_Ad/1 -> VESC_BrkPSetLe_MPa_sat/1
  VESC_BrkPSetLe_MPa_sat/1 -> VESC_BrkPSetLe_MPa_Out/1
  Demux/5 -> VESC_BrkPSetLe_MPa_Sub/1(In1)
  VESC_BrkPSetLe_MPa_Sub/1(Out1) -> VESC_BrkPSetLe_MPa_Convert/1
  VESC_BrkPSetLe_MPa_Convert/1 -> VESC_BrkPSetLe_MPa_L/1
  VESC_BrkPSetLe_MPa_L/1 -> VESC_BrkPSetLe_MPa_S/1
  VESC_BrkPSetLe_MPa_S/1 -> VESC_BrkPSetLe_MPacv/1
  VESC_BrkPSetLe_MPacv/1 -> VESC_BrkPSetLe_MPa_F/1
  VESC_BrkFlt_enum_F/1 -> VESC_BrkFlt_enum_Ad/1
  VESC_BrkFlt_enum_O/1 -> VESC_BrkFlt_enum_Ad/2
  VESC_BrkFlt_enum_Ad/1 -> VESC_BrkFlt_enum_sat/1
  VESC_BrkFlt_enum_sat/1 -> VESC_BrkFlt_enum_Out/1
  Demux/4 -> VESC_BrkFlt_enum_Sub/1(In1)
  VESC_BrkFlt_enum_Sub/1(Out1) -> VESC_BrkFlt_enum_Convert/1
  VESC_BrkFlt_enum_Convert/1 -> VESC_BrkFlt_enum_L/1
  VESC_BrkFlt_enum_L/1 -> VESC_BrkFlt_enum_S/1
  VESC_BrkFlt_enum_S/1 -> VESC_BrkFlt_enumcv/1
  VESC_BrkFlt_enumcv/1 -> VESC_BrkFlt_enum_F/1
  VESC_HotSts_flg_F/1 -> VESC_HotSts_flg_Ad/1
  VESC_HotSts_flg_O/1 -> VESC_HotSts_flg_Ad/2
  VESC_HotSts_flg_Ad/1 -> VESC_HotSts_flg_sat/1
  VESC_HotSts_flg_sat/1 -> VESC_HotSts_flg_Out/1
  Demux/3 -> VESC_BrkReq_flg_Sub/1(In1), VESC_ParkReq_flg_Sub/1(In1), VESC_HotSts_flg_Sub/1(In1)
  VESC_HotSts_flg_Sub/1(Out1) -> VESC_HotSts_flg_Convert/1
  VESC_HotSts_flg_Convert/1 -> VESC_HotSts_flg_L/1
  VESC_HotSts_flg_L/1 -> VESC_HotSts_flg_S/1
  VESC_HotSts_flg_S/1 -> VESC_HotSts_flgcv/1
  VESC_HotSts_flgcv/1 -> VESC_HotSts_flg_F/1
  VESC_BrkReq_flg_F/1 -> VESC_BrkReq_flg_Ad/1
  VESC_BrkReq_flg_O/1 -> VESC_BrkReq_flg_Ad/2
  VESC_BrkReq_flg_Ad/1 -> VESC_BrkReq_flg_sat/1
  VESC_BrkReq_flg_sat/1 -> VESC_BrkReq_flg_Out/1
  VESC_BrkReq_flg_Sub/1(Out1) -> VESC_BrkReq_flg_Convert/1
  VESC_BrkReq_flg_Convert/1 -> VESC_BrkReq_flg_L/1
  VESC_BrkReq_flg_L/1 -> VESC_BrkReq_flg_S/1
  VESC_BrkReq_flg_S/1 -> VESC_BrkReq_flgcv/1
  VESC_BrkReq_flgcv/1 -> VESC_BrkReq_flg_F/1
  VESC_ParkReq_flg_F/1 -> VESC_ParkReq_flg_Ad/1
  VESC_ParkReq_flg_O/1 -> VESC_ParkReq_flg_Ad/2
  VESC_ParkReq_flg_Ad/1 -> VESC_ParkReq_flg_sat/1
  VESC_ParkReq_flg_sat/1 -> VESC_ParkReq_flg_Out/1
  VESC_ParkReq_flg_Sub/1(Out1) -> VESC_ParkReq_flg_Convert/1
  VESC_ParkReq_flg_Convert/1 -> VESC_ParkReq_flg_L/1
  VESC_ParkReq_flg_L/1 -> VESC_ParkReq_flg_S/1
  VESC_ParkReq_flg_S/1 -> VESC_ParkReq_flgcv/1
  VESC_ParkReq_flgcv/1 -> VESC_ParkReq_flg_F/1
  VESC_BrkPRi_MPa_F/1 -> VESC_BrkPRi_MPa_Ad/1
  VESC_BrkPRi_MPa_O/1 -> VESC_BrkPRi_MPa_Ad/2
  VESC_BrkPRi_MPa_Ad/1 -> VESC_BrkPRi_MPa_sat/1
  VESC_BrkPRi_MPa_sat/1 -> VESC_BrkPRi_MPa_Out/1
  Demux/2 -> VESC_BrkPRi_MPa_Sub/1(In1)
  VESC_BrkPRi_MPa_Sub/1(Out1) -> VESC_BrkPRi_MPa_Convert/1
  VESC_BrkPRi_MPa_Convert/1 -> VESC_BrkPRi_MPa_L/1
  VESC_BrkPRi_MPa_L/1 -> VESC_BrkPRi_MPa_S/1
  VESC_BrkPRi_MPa_S/1 -> VESC_BrkPRi_MPacv/1
  VESC_BrkPRi_MPacv/1 -> VESC_BrkPRi_MPa_F/1
  VESC_BrkPLe_MPa_F/1 -> VESC_BrkPLe_MPa_Ad/1
  VESC_BrkPLe_MPa_O/1 -> VESC_BrkPLe_MPa_Ad/2
  VESC_BrkPLe_MPa_Ad/1 -> VESC_BrkPLe_MPa_sat/1
  VESC_BrkPLe_MPa_sat/1 -> VESC_BrkPLe_MPa_Out/1
  Demux/1 -> VESC_BrkPLe_MPa_Sub/1(In1)
  VESC_BrkPLe_MPa_Sub/1(Out1) -> VESC_BrkPLe_MPa_Convert/1
  VESC_BrkPLe_MPa_Convert/1 -> VESC_BrkPLe_MPa_L/1
  VESC_BrkPLe_MPa_L/1 -> VESC_BrkPLe_MPa_S/1
  VESC_BrkPLe_MPa_S/1 -> VESC_BrkPLe_MPacv/1
  VESC_BrkPLe_MPacv/1 -> VESC_BrkPLe_MPa_F/1
  input/1 -> Demux/1

== system DDCU_wxt_v02_forA_LabviewV02/Data_Input/HCU1_VCU/HCU1_VCU ==
  input : Inport
  Enable : EnablePort
  Demux : Demux  Outputs=8
  acc_Ad : Sum
  acc_Convert : DataTypeConversion  OutDataTypeStr=uint32
  acc_F : Gain
  acc_L : simulink/Logic and Bit Operations/Bitwise Operator  logicop=AND  UseBitMask=on  BitMask=65535  BitMaskRealWorld=Stored Integer
  acc_O : Constant  Value=0  OutDataTypeStr=single
  acc_S : ArithShift
  acc_Sub : Subsystem
  acc_sat : Saturate  UpperLimit=65535  LowerLimit=0
  acccv : DataTypeConversion
  accinput2_Ad : Sum
  accinput2_C : Constant  Value=256
  accinput2_P : Product
  break_Ad : Sum
  break_Convert : DataTypeConversion  OutDataTypeStr=uint32
  break_F : Gain
  break_L : simulink/Logic and Bit Operations/Bitwise Operator  logicop=AND  UseBitMask=on  BitMask=255  BitMaskRealWorld=Stored Integer
  break_O : Constant  Value=0  OutDataTypeStr=single
  break_S : ArithShift
  break_Sub : Subsystem
  break_sat : Saturate  UpperLimit=255  LowerLimit=0
  breakcv : DataTypeConversion
  pwr_limit_Ad : Sum
  pwr_limit_Convert : DataTypeConversion  OutDataTypeStr=uint32
  pwr_limit_F : Gain
  pwr_limit_L : simulink/Logic and Bit Operations/Bitwise Operator  logicop=AND  UseBitMask=on  BitMask=255  BitMaskRealWorld=Stored Integer
  pwr_limit_O : Constant  Value=0  OutDataTypeStr=single
  pwr_limit_S : ArithShift
  pwr_limit_Sub : Subsystem
  pwr_limit_sat : Saturate  UpperLimit=255  LowerLimit=0
  pwr_limitcv : DataTypeConversion
  real_velocity_Ad : Sum
  real_velocity_Convert : DataTypeConversion  OutDataTypeStr=uint32
  real_velocity_F : Gain
  real_velocity_L : simulink/Logic and Bit Operations/Bitwise Operator  logicop=AND  UseBitMask=on  BitMask=255  BitMaskRealWorld=Stored Integer
  real_velocity_O : Constant  Value=0  OutDataTypeStr=single
  real_velocity_S : ArithShift
  real_velocity_Sub : Subsystem
  real_velocity_sat : Saturate  UpperLimit=255  LowerLimit=0
  real_velocitycv : DataTypeConversion
  turn_Ad : Sum
  turn_Convert : DataTypeConversion  OutDataTypeStr=uint32
  turn_F : Gain
  turn_L : simulink/Logic and Bit Operations/Bitwise Operator  logicop=AND  UseBitMask=on  BitMask=65535  BitMaskRealWorld=Stored Integer
  turn_O : Constant  Value=0  OutDataTypeStr=single
  turn_S : ArithShift
  turn_Sub : Subsystem
  turn_sat : Saturate  UpperLimit=65535  LowerLimit=0
  turncv : DataTypeConversion
  turninput4_Ad : Sum
  turninput4_C : Constant  Value=256
  turninput4_P : Product
  turn_Out : Outport
  real_velocity_Out : Outport  Port=2
  pwr_limit_Out : Outport  Port=3
  break_Out : Outport  Port=4
  acc_Out : Outport  Port=5
  wires:
  turn_F/1 -> turn_Ad/1
  turn_O/1 -> turn_Ad/2
  turn_Ad/1 -> turn_sat/1
  turn_sat/1 -> turn_Out/1
  Demux/4 -> turninput4_P/1
  turninput4_C/1 -> turninput4_P/2
  turninput4_P/1 -> turninput4_Ad/1
  Demux/3 -> turninput4_Ad/2
  turninput4_Ad/1 -> turn_Sub/1(In1)
  turn_Sub/1(Out1) -> turn_Convert/1
  turn_Convert/1 -> turn_L/1
  turn_L/1 -> turn_S/1
  turn_S/1 -> turncv/1
  turncv/1 -> turn_F/1
  real_velocity_F/1 -> real_velocity_Ad/1
  real_velocity_O/1 -> real_velocity_Ad/2
  real_velocity_Ad/1 -> real_velocity_sat/1
  real_velocity_sat/1 -> real_velocity_Out/1
  Demux/5 -> real_velocity_Sub/1(In1)
  real_velocity_Sub/1(Out1) -> real_velocity_Convert/1
  real_velocity_Convert/1 -> real_velocity_L/1
  real_velocity_L/1 -> real_velocity_S/1
  real_velocity_S/1 -> real_velocitycv/1
  real_velocitycv/1 -> real_velocity_F/1
  pwr_limit_F/1 -> pwr_limit_Ad/1
  pwr_limit_O/1 -> pwr_limit_Ad/2
  pwr_limit_Ad/1 -> pwr_limit_sat/1
  pwr_limit_sat/1 -> pwr_limit_Out/1
  Demux/6 -> pwr_limit_Sub/1(In1)
  pwr_limit_Sub/1(Out1) -> pwr_limit_Convert/1
  pwr_limit_Convert/1 -> pwr_limit_L/1
  pwr_limit_L/1 -> pwr_limit_S/1
  pwr_limit_S/1 -> pwr_limitcv/1
  pwr_limitcv/1 -> pwr_limit_F/1
  break_F/1 -> break_Ad/1
  break_O/1 -> break_Ad/2
  break_Ad/1 -> break_sat/1
  break_sat/1 -> break_Out/1
  Demux/7 -> break_Sub/1(In1)
  break_Sub/1(Out1) -> break_Convert/1
  break_Convert/1 -> break_L/1
  break_L/1 -> break_S/1
  break_S/1 -> breakcv/1
  breakcv/1 -> break_F/1
  acc_F/1 -> acc_Ad/1
  acc_O/1 -> acc_Ad/2
  acc_Ad/1 -> acc_sat/1
  acc_sat/1 -> acc_Out/1
  Demux/2 -> accinput2_P/1
  accinput2_C/1 -> accinput2_P/2
  accinput2_P/1 -> accinput2_Ad/1
  Demux/1 -> accinput2_Ad/2
  accinput2_Ad/1 -> acc_Sub/1(In1)
  acc_Sub/1(Out1) -> acc_Convert/1
  acc_Convert/1 -> acc_L/1
  acc_L/1 -> acc_S/1
  acc_S/1 -> acccv/1
  acccv/1 -> acc_F/1
  input/1 -> Demux/1

== system DDCU_wxt_v02_forA_LabviewV02/Data_Input/HCU1_VCU1/MUC1_VCU1 ==
  input : Inport
  Enable : EnablePort
  Demux : Demux  Outputs=8
  spd_mot_lf_Ad : Sum
  spd_mot_lf_Convert : DataTypeConversion  OutDataTypeStr=uint32
  spd_mot_lf_F : Gain
  spd_mot_lf_L : simulink/Logic and Bit Operations/Bitwise Operator  logicop=AND  UseBitMask=on  BitMask=65535  BitMaskRealWorld=Stored Integer
  spd_mot_lf_O : Constant  Value=0  OutDataTypeStr=single
  spd_mot_lf_S : ArithShift
  spd_mot_lf_Sub : Subsystem
  spd_mot_lf_sat : Saturate  UpperLimit=65535  LowerLimit=0
  spd_mot_lfcv : DataTypeConversion
  spd_mot_lfinput6_Ad : Sum
  spd_mot_lfinput6_C : Constant  Value=256
  spd_mot_lfinput6_P : Product
  spd_mot_lr_Ad : Sum
  spd_mot_lr_Convert : DataTypeConversion  OutDataTypeStr=uint32
  spd_mot_lr_F : Gain
  spd_mot_lr_L : simulink/Logic and Bit Operations/Bitwise Operator  logicop=AND  UseBitMask=on  BitMask=65535  BitMaskRealWorld=Stored Integer
  spd_mot_lr_O : Constant  Value=0  OutDataTypeStr=single
  spd_mot_lr_S : ArithShift
  spd_mot_lr_Sub : Subsystem
  spd_mot_lr_sat : Saturate  UpperLimit=65535  LowerLimit=0
  spd_mot_lrcv : DataTypeConversion
  spd_mot_lrinput8_Ad : Sum
  spd_mot_lrinput8_C : Constant  Value=256
  spd_mot_lrinput8_P : Product
  spd_mot_rf_Ad : Sum
  spd_mot_rf_Convert : DataTypeConversion  OutDataTypeStr=uint32
  spd_mot_rf_F : Gain
  spd_mot_rf_L : simulink/Logic and Bit Operations/Bitwise Operator  logicop=AND  UseBitMask=on  BitMask=65535  BitMaskRealWorld=Stored Integer
  spd_mot_rf_O : Constant  Value=0  OutDataTypeStr=single
  spd_mot_rf_S : ArithShift
  spd_mot_rf_Sub : Subsystem
  spd_mot_rf_sat : Saturate  UpperLimit=65535  LowerLimit=0
  spd_mot_rfcv : DataTypeConversion
  spd_mot_rfinput2_Ad : Sum
  spd_mot_rfinput2_C : Constant  Value=256
  spd_mot_rfinput2_P : Product
  spd_mot_rr_Ad : Sum
  spd_mot_rr_Convert : DataTypeConversion  OutDataTypeStr=uint32
  spd_mot_rr_F : Gain
  spd_mot_rr_L : simulink/Logic and Bit Operations/Bitwise Operator  logicop=AND  UseBitMask=on  BitMask=65535  BitMaskRealWorld=Stored Integer
  spd_mot_rr_O : Constant  Value=0  OutDataTypeStr=single
  spd_mot_rr_S : ArithShift
  spd_mot_rr_Sub : Subsystem
  spd_mot_rr_sat : Saturate  UpperLimit=65535  LowerLimit=0
  spd_mot_rrcv : DataTypeConversion
  spd_mot_rrinput4_Ad : Sum
  spd_mot_rrinput4_C : Constant  Value=256
  spd_mot_rrinput4_P : Product
  spd_mot_rr_Out : Outport
  spd_mot_rf_Out : Outport  Port=2
  spd_mot_lr_Out : Outport  Port=3
  spd_mot_lf_Out : Outport  Port=4
  wires:
  spd_mot_rr_F/1 -> spd_mot_rr_Ad/1
  spd_mot_rr_O/1 -> spd_mot_rr_Ad/2
  spd_mot_rr_Ad/1 -> spd_mot_rr_sat/1
  spd_mot_rr_sat/1 -> spd_mot_rr_Out/1
  Demux/4 -> spd_mot_rrinput4_P/1
  spd_mot_rrinput4_C/1 -> spd_mot_rrinput4_P/2
  spd_mot_rrinput4_P/1 -> spd_mot_rrinput4_Ad/1
  Demux/3 -> spd_mot_rrinput4_Ad/2
  spd_mot_rrinput4_Ad/1 -> spd_mot_rr_Sub/1(In1)
  spd_mot_rr_Sub/1(Out1) -> spd_mot_rr_Convert/1
  spd_mot_rr_Convert/1 -> spd_mot_rr_L/1
  spd_mot_rr_L/1 -> spd_mot_rr_S/1
  spd_mot_rr_S/1 -> spd_mot_rrcv/1
  spd_mot_rrcv/1 -> spd_mot_rr_F/1
  spd_mot_rf_F/1 -> spd_mot_rf_Ad/1
  spd_mot_rf_O/1 -> spd_mot_rf_Ad/2
  spd_mot_rf_Ad/1 -> spd_mot_rf_sat/1
  spd_mot_rf_sat/1 -> spd_mot_rf_Out/1
  Demux/2 -> spd_mot_rfinput2_P/1
  spd_mot_rfinput2_C/1 -> spd_mot_rfinput2_P/2
  spd_mot_rfinput2_P/1 -> spd_mot_rfinput2_Ad/1
  Demux/1 -> spd_mot_rfinput2_Ad/2
  spd_mot_rfinput2_Ad/1 -> spd_mot_rf_Sub/1(In1)
  spd_mot_rf_Sub/1(Out1) -> spd_mot_rf_Convert/1
  spd_mot_rf_Convert/1 -> spd_mot_rf_L/1
  spd_mot_rf_L/1 -> spd_mot_rf_S/1
  spd_mot_rf_S/1 -> spd_mot_rfcv/1
  spd_mot_rfcv/1 -> spd_mot_rf_F/1
  spd_mot_lr_F/1 -> spd_mot_lr_Ad/1
  spd_mot_lr_O/1 -> spd_mot_lr_Ad/2
  spd_mot_lr_Ad/1 -> spd_mot_lr_sat/1
  spd_mot_lr_sat/1 -> spd_mot_lr_Out/1
  Demux/8 -> spd_mot_lrinput8_P/1
  spd_mot_lrinput8_C/1 -> spd_mot_lrinput8_P/2
  spd_mot_lrinput8_P/1 -> spd_mot_lrinput8_Ad/1
  Demux/7 -> spd_mot_lrinput8_Ad/2
  spd_mot_lrinput8_Ad/1 -> spd_mot_lr_Sub/1(In1)
  spd_mot_lr_Sub/1(Out1) -> spd_mot_lr_Convert/1
  spd_mot_lr_Convert/1 -> spd_mot_lr_L/1
  spd_mot_lr_L/1 -> spd_mot_lr_S/1
  spd_mot_lr_S/1 -> spd_mot_lrcv/1
  spd_mot_lrcv/1 -> spd_mot_lr_F/1
  spd_mot_lf_F/1 -> spd_mot_lf_Ad/1
  spd_mot_lf_O/1 -> spd_mot_lf_Ad/2
  spd_mot_lf_Ad/1 -> spd_mot_lf_sat/1
  spd_mot_lf_sat/1 -> spd_mot_lf_Out/1
  Demux/6 -> spd_mot_lfinput6_P/1
  spd_mot_lfinput6_C/1 -> spd_mot_lfinput6_P/2
  spd_mot_lfinput6_P/1 -> spd_mot_lfinput6_Ad/1
  Demux/5 -> spd_mot_lfinput6_Ad/2
  spd_mot_lfinput6_Ad/1 -> spd_mot_lf_Sub/1(In1)
  spd_mot_lf_Sub/1(Out1) -> spd_mot_lf_Convert/1
  spd_mot_lf_Convert/1 -> spd_mot_lf_L/1
  spd_mot_lf_L/1 -> spd_mot_lf_S/1
  spd_mot_lf_S/1 -> spd_mot_lfcv/1
  spd_mot_lfcv/1 -> spd_mot_lf_F/1
  input/1 -> Demux/1

== system DDCU_wxt_v02_forA_LabviewV02/Data_Input/HCU2_VCU/HCU2_VCU ==
  input : Inport
  Enable : EnablePort
  Demux : Demux  Outputs=8
  daodang_Ad : Sum
  daodang_Convert : DataTypeConversion  OutDataTypeStr=uint32
  daodang_F : Gain
  daodang_L : simulink/Logic and Bit Operations/Bitwise Operator  logicop=AND  UseBitMask=on  BitMask=4  BitMaskRealWorld=Stored Integer
  daodang_O : Constant  Value=0  OutDataTypeStr=single
  daodang_S : ArithShift  BitShiftNumber=2
  daodang_Sub : Subsystem
  daodang_sat : Saturate  UpperLimit=1  LowerLimit=0
  daodangcv : DataTypeConversion
  kongdang_Ad : Sum
  kongdang_Convert : DataTypeConversion  OutDataTypeStr=uint32
  kongdang_F : Gain
  kongdang_L : simulink/Logic and Bit Operations/Bitwise Operator  logicop=AND  UseBitMask=on  BitMask=2  BitMaskRealWorld=Stored Integer
  kongdang_O : Constant  Value=0  OutDataTypeStr=single
  kongdang_S : ArithShift  BitShiftNumber=1
  kongdang_Sub : Subsystem
  kongdang_sat : Saturate  UpperLimit=1  LowerLimit=0
  kongdangcv : DataTypeConversion
  qianjin_Ad : Sum
  qianjin_Convert : DataTypeConversion  OutDataTypeStr=uint32
  qianjin_F : Gain
  qianjin_L : simulink/Logic and Bit Operations/Bitwise Operator  logicop=AND  UseBitMask=on  BitMask=1  BitMaskRealWorld=Stored Integer
  qianjin_O : Constant  Value=0  OutDataTypeStr=single
  qianjin_S : ArithShift
  qianjin_Sub : Subsystem
  qianjin_sat : Saturate  UpperLimit=1  LowerLimit=0
  qianjincv : DataTypeConversion
  zhongxinzhuanxiang_Ad : Sum
  zhongxinzhuanxiang_Convert : DataTypeConversion  OutDataTypeStr=uint32
  zhongxinzhuanxiang_F : Gain
  zhongxinzhuanxiang_L : simulink/Logic and Bit Operations/Bitwise Operator  logicop=AND  UseBitMask=on  BitMask=8  BitMaskRealWorld=Stored Integer
  zhongxinzhuanxiang_O : Constant  Value=0  OutDataTypeStr=single
  zhongxinzhuanxiang_S : ArithShift  BitShiftNumber=3
  zhongxinzhuanxiang_Sub : Subsystem
  zhongxinzhuanxiang_sat : Saturate  UpperLimit=1  LowerLimit=0
  zhongxinzhuanxiangcv : DataTypeConversion
  zhuche_Ad : Sum
  zhuche_Convert : DataTypeConversion  OutDataTypeStr=uint32
  zhuche_F : Gain
  zhuche_L : simulink/Logic and Bit Operations/Bitwise Operator  logicop=AND  UseBitMask=on  BitMask=16  BitMaskRealWorld=Stored Integer
  zhuche_O : Constant  Value=0  OutDataTypeStr=single
  zhuche_S : ArithShift  BitShiftNumber=4
  zhuche_Sub : Subsystem
  zhuche_sat : Saturate  UpperLimit=1  LowerLimit=0
  zhuchecv : DataTypeConversion
  zhuche_Out : Outport
  zhongxinzhuanxiang_Out : Outport  Port=2
  qianjin_Out : Outport  Port=3
  kongdang_Out : Outport  Port=4
  daodang_Out : Outport  Port=5
  wires:
  zhuche_F/1 -> zhuche_Ad/1
  zhuche_O/1 -> zhuche_Ad/2
  zhuche_Ad/1 -> zhuche_sat/1
  zhuche_sat/1 -> zhuche_Out/1
  Demux/1 -> qianjin_Sub/1(In1), daodang_Sub/1(In1), zhongxinzhuanxiang_Sub/1(In1), zhuche_Sub/1(In1), kongdang_Sub/1(In1)
  zhuche_Sub/1(Out1) -> zhuche_Convert/1
  zhuche_Convert/1 -> zhuche_L/1
  zhuche_L/1 -> zhuche_S/1
  zhuche_S/1 -> zhuchecv/1
  zhuchecv/1 -> zhuche_F/1
  zhongxinzhuanxiang_F/1 -> zhongxinzhuanxiang_Ad/1
  zhongxinzhuanxiang_O/1 -> zhongxinzhuanxiang_Ad/2
  zhongxinzhuanxiang_Ad/1 -> zhongxinzhuanxiang_sat/1
  zhongxinzhuanxiang_sat/1 -> zhongxinzhuanxiang_Out/1
  zhongxinzhuanxiang_Sub/1(Out1) -> zhongxinzhuanxiang_Convert/1
  zhongxinzhuanxiang_Convert/1 -> zhongxinzhuanxiang_L/1
  zhongxinzhuanxiang_L/1 -> zhongxinzhuanxiang_S/1
  zhongxinzhuanxiang_S/1 -> zhongxinzhuanxiangcv/1
  zhongxinzhuanxiangcv/1 -> zhongxinzhuanxiang_F/1
  qianjin_F/1 -> qianjin_Ad/1
  qianjin_O/1 -> qianjin_Ad/2
  qianjin_Ad/1 -> qianjin_sat/1
  qianjin_sat/1 -> qianjin_Out/1
  qianjin_Sub/1(Out1) -> qianjin_Convert/1
  qianjin_Convert/1 -> qianjin_L/1
  qianjin_L/1 -> qianjin_S/1
  qianjin_S/1 -> qianjincv/1
  qianjincv/1 -> qianjin_F/1
  kongdang_F/1 -> kongdang_Ad/1
  kongdang_O/1 -> kongdang_Ad/2
  kongdang_Ad/1 -> kongdang_sat/1
  kongdang_sat/1 -> kongdang_Out/1
  kongdang_Sub/1(Out1) -> kongdang_Convert/1
  kongdang_Convert/1 -> kongdang_L/1
  kongdang_L/1 -> kongdang_S/1
  kongdang_S/1 -> kongdangcv/1
  kongdangcv/1 -> kongdang_F/1
  daodang_F/1 -> daodang_Ad/1
  daodang_O/1 -> daodang_Ad/2
  daodang_Ad/1 -> daodang_sat/1
  daodang_sat/1 -> daodang_Out/1
  daodang_Sub/1(Out1) -> daodang_Convert/1
  daodang_Convert/1 -> daodang_L/1
  daodang_L/1 -> daodang_S/1
  daodang_S/1 -> daodangcv/1
  daodangcv/1 -> daodang_F/1
  input/1 -> Demux/1
